simulink model "SimpleModel"  (R2017a)
settings: Solver=VariableStepAuto  StartTime=0.0  StopTime=100  RelTol=1e-3
settings Model: Creator=GusBus  LastModifiedBy=GusBus

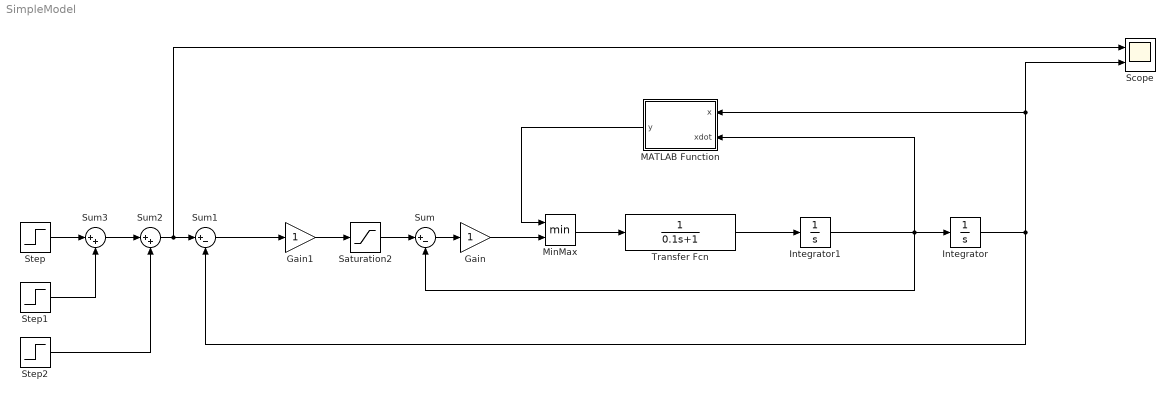
== system SimpleModel ==
  Gain : Gain
  Gain1 : Gain
  Integrator : Integrator
  Integrator1 : Integrator
  MATLAB Function : MATLAB Function  TreatAsAtomicUnit=on
  MinMax : MinMax  Inputs=2
  Saturation2 : Saturate  UpperLimit=2  LowerLimit=-2
  Scope : Scope  NumInputPorts=2
  Step : Step  After=4  SampleTime=0
  Step1 : Step  Time=20  After=6  SampleTime=0
  Step2 : Step  Time=50  After=-8  SampleTime=0
  Sum : Sum  Inputs=|+-
  Sum1 : Sum  Inputs=|+-
  Sum2 : Sum  Inputs=|++
  Sum3 : Sum  Inputs=|++
  Transfer Fcn : TransferFcn  Denominator=[0.1 1]
  wires:
  Step/1 -> Sum3/1
  Step1/1 -> Sum3/2
  Integrator1/1 -> Sum/2, Integrator/1, MATLAB Function/2(xdot)
  Step2/1 -> Sum2/2
  Saturation2/1 -> Sum/1
  MinMax/1 -> Transfer Fcn/1
  Sum/1 -> Gain/1
  MATLAB Function/1(y) -> MinMax/1
  Transfer Fcn/1 -> Integrator1/1
  Sum2/1 -> Scope/1, Sum1/1
  Integrator/1 -> Sum1/2, MATLAB Function/1(x), Scope/2
  Gain/1 -> MinMax/2
  Sum1/1 -> Gain1/1
  Sum3/1 -> Sum2/1
  Gain1/1 -> Saturation2/1

== matlab function SimpleModel/MATLAB Function ==
  data: x input; y output; xdot input
function y = fcn(x,xdot)

y = 10*(5-x)-10*xdot;
